simulink model "test1"  (R2018b)
settings: Solver=VariableStepAuto  StartTime=0.0  StopTime=10.0  RelTol=1e-3
settings Model: Creator=ruty  LastModifiedBy=ruty

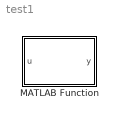
== system test1 ==
  MATLAB Function : MATLAB Function  TreatAsAtomicUnit=on

== matlab function test1/MATLAB Function ==
  data: u input; y output
function y = fcn(u)

y = u;
